simulink model "WatermelonProj"  (R2021b)
settings: Solver=VariableStepAuto  StartTime=0.0  StopTime=25000  RelTol=1e-3
settings Model: Creator=ammo5  LastModifiedBy=ammo5

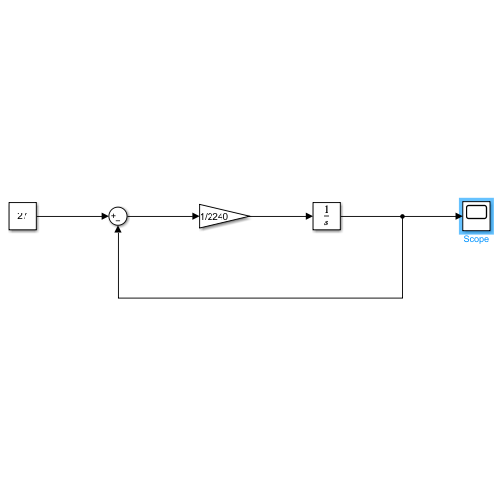
[thumbnail: Simulink's stored preview of the top-level diagram]
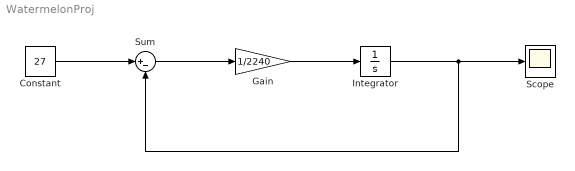
== system WatermelonProj ==
  Constant : Constant  Value=27
  Gain : Gain  Gain=1/2240
  Integrator : Integrator  InitialCondition=5
  Scope : Scope
  Sum : Sum  Inputs=|+-
  wires:
  Constant/1 -> Sum/1
  Sum/1 -> Gain/1
  Gain/1 -> Integrator/1
  Integrator/1 -> Sum/2, Scope/1
